simulink model "gm_uz_pmsm_model_9ph_vnl"  (R2021a)
settings: Solver=FixedStepAuto  StartTime=0.0  StopTime=.5  RelTol=1e-3
PreLoadFcn:
  | uz_pmsm_model_init_parameter
undefined symbols (not defined in the file or in its folder): c, friction_coefficient, inertia, k_i_d, k_p_d, k_p_q, L_d, L_o1, L_o2, L_q, L_x1, L_x2, L_y1, L_y2, L_zero, polepair, psi_pm, R_1, static_friction_torque, ts
libraries: hdlmdlgenlib x220, hdlsllib x18, simulink x11, pid_lib x2
(part 4 of 4)

== system gm_uz_pmsm_model_9ph_vnl/uz_pmsm_model_9ph/Transformation/Divide2 ==
  In1 : Inport
  In2 : Inport  Port=2
  Divide2 : Product  Inputs=**  OutDataTypeStr=single  SampleTime=1e-08
  Out1 : Outport
  wires:
  Divide2/1 -> Out1/1
  In2/1 -> Divide2/2
  In1/1 -> Divide2/1

== system gm_uz_pmsm_model_9ph_vnl/uz_pmsm_model_9ph/Transformation/Divide3 ==
  In1 : Inport
  In2 : Inport  Port=2
  Divide3 : Product  Inputs=**  OutDataTypeStr=single  SampleTime=1e-08
  Out1 : Outport
  wires:
  Divide3/1 -> Out1/1
  In2/1 -> Divide3/2
  In1/1 -> Divide3/1

== system gm_uz_pmsm_model_9ph_vnl/uz_pmsm_model_9ph/Transformation/Transformation_MAC ==
  in0 : Inport  OutDataTypeStr=fixdt(1, 18, 19)  PortDimensions=[9 1]  SampleTime=1e-08
  in1 : Inport  Port=2  OutDataTypeStr=fixdt(1, 25, 12)  PortDimensions=[9]  SampleTime=1e-08
  globalSchedule : EnablePort  OutDataTypeStr=boolean
  PipelineRegister : Delay  DelayLength=double(8)  InitialCondition=0
  t : hdlsllib/HDL Operations/Multiply-Accumulate  opMode=Vector  initValueSetting=Dialog  initValue=0  initValueSetting2=Dialog  initValue2=0  initValueSetting3=Dialog  initValue3=0  num_samples=2  RndMeth2=Floor  RndMeth3=Floor  OutDataTypeStr=fixdt(1, 43, 31)  datatype2=Inherit: Inherit via back propagation  datatype3=Inherit: Inherit via back propagation  validOut=on  endInandOut=on  startOut=on  countOut=on  dim=-1  DoSatur=off  parallel=off
      settings: SourceProductBaseCode=SL
  out0 : Outport  OutDataTypeStr=fixdt(1, 43, 31)  SampleTime=1e-08  InitialOutput=0
  wires:
  t/1 -> PipelineRegister/1
  in1/1 -> t/2
  in0/1 -> t/1
  PipelineRegister/1 -> out0/1

== system gm_uz_pmsm_model_9ph_vnl/uz_pmsm_model_9ph/Transformation/Transformation_MAC1 ==
  in0 : Inport  OutDataTypeStr=fixdt(1, 18, 19)  PortDimensions=[9 1]  SampleTime=1e-08
  in1 : Inport  Port=2  OutDataTypeStr=fixdt(1, 25, 12)  PortDimensions=[9]  SampleTime=1e-08
  globalSchedule : EnablePort  OutDataTypeStr=boolean
  PipelineRegister : Delay  DelayLength=double(8)  InitialCondition=0
  t : hdlsllib/HDL Operations/Multiply-Accumulate  opMode=Vector  initValueSetting=Dialog  initValue=0  initValueSetting2=Dialog  initValue2=0  initValueSetting3=Dialog  initValue3=0  num_samples=2  RndMeth2=Floor  RndMeth3=Floor  OutDataTypeStr=fixdt(1, 43, 31)  datatype2=Inherit: Inherit via back propagation  datatype3=Inherit: Inherit via back propagation  validOut=on  endInandOut=on  startOut=on  countOut=on  dim=-1  DoSatur=off  parallel=off
      settings: SourceProductBaseCode=SL
  out0 : Outport  OutDataTypeStr=fixdt(1, 43, 31)  SampleTime=1e-08  InitialOutput=0
  wires:
  t/1 -> PipelineRegister/1
  in1/1 -> t/2
  in0/1 -> t/1
  PipelineRegister/1 -> out0/1

== system gm_uz_pmsm_model_9ph_vnl/uz_pmsm_model_9ph/Transformation/Transformation_MAC2 ==
  in0 : Inport  OutDataTypeStr=fixdt(1, 18, 19)  PortDimensions=[9 1]  SampleTime=1e-08
  in1 : Inport  Port=2  OutDataTypeStr=fixdt(1, 25, 12)  PortDimensions=[9]  SampleTime=1e-08
  globalSchedule : EnablePort  OutDataTypeStr=boolean
  PipelineRegister : Delay  DelayLength=double(8)  InitialCondition=0
  t : hdlsllib/HDL Operations/Multiply-Accumulate  opMode=Vector  initValueSetting=Dialog  initValue=0  initValueSetting2=Dialog  initValue2=0  initValueSetting3=Dialog  initValue3=0  num_samples=2  RndMeth2=Floor  RndMeth3=Floor  OutDataTypeStr=fixdt(1, 43, 31)  datatype2=Inherit: Inherit via back propagation  datatype3=Inherit: Inherit via back propagation  validOut=on  endInandOut=on  startOut=on  countOut=on  dim=-1  DoSatur=off  parallel=off
      settings: SourceProductBaseCode=SL
  out0 : Outport  OutDataTypeStr=fixdt(1, 43, 31)  SampleTime=1e-08  InitialOutput=0
  wires:
  t/1 -> PipelineRegister/1
  in1/1 -> t/2
  in0/1 -> t/1
  PipelineRegister/1 -> out0/1

== system gm_uz_pmsm_model_9ph_vnl/uz_pmsm_model_9ph/Transformation/Transformation_MAC3 ==
  in0 : Inport  OutDataTypeStr=fixdt(1, 18, 19)  PortDimensions=[9 1]  SampleTime=1e-08
  in1 : Inport  Port=2  OutDataTypeStr=fixdt(1, 25, 12)  PortDimensions=[9]  SampleTime=1e-08
  globalSchedule : EnablePort  OutDataTypeStr=boolean
  PipelineRegister : Delay  DelayLength=double(8)  InitialCondition=0
  t : hdlsllib/HDL Operations/Multiply-Accumulate  opMode=Vector  initValueSetting=Dialog  initValue=0  initValueSetting2=Dialog  initValue2=0  initValueSetting3=Dialog  initValue3=0  num_samples=2  RndMeth2=Floor  RndMeth3=Floor  OutDataTypeStr=fixdt(1, 43, 31)  datatype2=Inherit: Inherit via back propagation  datatype3=Inherit: Inherit via back propagation  validOut=on  endInandOut=on  startOut=on  countOut=on  dim=-1  DoSatur=off  parallel=off
      settings: SourceProductBaseCode=SL
  out0 : Outport  OutDataTypeStr=fixdt(1, 43, 31)  SampleTime=1e-08  InitialOutput=0
  wires:
  t/1 -> PipelineRegister/1
  in1/1 -> t/2
  in0/1 -> t/1
  PipelineRegister/1 -> out0/1

== system gm_uz_pmsm_model_9ph_vnl/uz_pmsm_model_9ph/Transformation/Transformation_MAC4 ==
  in0 : Inport  OutDataTypeStr=fixdt(1, 18, 19)  PortDimensions=[9 1]  SampleTime=1e-08
  in1 : Inport  Port=2  OutDataTypeStr=fixdt(1, 25, 12)  PortDimensions=[9]  SampleTime=1e-08
  globalSchedule : EnablePort  OutDataTypeStr=boolean
  PipelineRegister : Delay  DelayLength=double(8)  InitialCondition=0
  t : hdlsllib/HDL Operations/Multiply-Accumulate  opMode=Vector  initValueSetting=Dialog  initValue=0  initValueSetting2=Dialog  initValue2=0  initValueSetting3=Dialog  initValue3=0  num_samples=2  RndMeth2=Floor  RndMeth3=Floor  OutDataTypeStr=fixdt(1, 43, 31)  datatype2=Inherit: Inherit via back propagation  datatype3=Inherit: Inherit via back propagation  validOut=on  endInandOut=on  startOut=on  countOut=on  dim=-1  DoSatur=off  parallel=off
      settings: SourceProductBaseCode=SL
  out0 : Outport  OutDataTypeStr=fixdt(1, 43, 31)  SampleTime=1e-08  InitialOutput=0
  wires:
  t/1 -> PipelineRegister/1
  in1/1 -> t/2
  in0/1 -> t/1
  PipelineRegister/1 -> out0/1

== system gm_uz_pmsm_model_9ph_vnl/uz_pmsm_model_9ph/Transformation/Transformation_MAC5 ==
  in0 : Inport  OutDataTypeStr=fixdt(1, 18, 19)  PortDimensions=[9 1]  SampleTime=1e-08
  in1 : Inport  Port=2  OutDataTypeStr=fixdt(1, 25, 12)  PortDimensions=[9]  SampleTime=1e-08
  globalSchedule : EnablePort  OutDataTypeStr=boolean
  PipelineRegister : Delay  DelayLength=double(8)  InitialCondition=0
  t : hdlsllib/HDL Operations/Multiply-Accumulate  opMode=Vector  initValueSetting=Dialog  initValue=0  initValueSetting2=Dialog  initValue2=0  initValueSetting3=Dialog  initValue3=0  num_samples=2  RndMeth2=Floor  RndMeth3=Floor  OutDataTypeStr=fixdt(1, 43, 31)  datatype2=Inherit: Inherit via back propagation  datatype3=Inherit: Inherit via back propagation  validOut=on  endInandOut=on  startOut=on  countOut=on  dim=-1  DoSatur=off  parallel=off
      settings: SourceProductBaseCode=SL
  out0 : Outport  OutDataTypeStr=fixdt(1, 43, 31)  SampleTime=1e-08  InitialOutput=0
  wires:
  t/1 -> PipelineRegister/1
  in1/1 -> t/2
  in0/1 -> t/1
  PipelineRegister/1 -> out0/1

== system gm_uz_pmsm_model_9ph_vnl/uz_pmsm_model_9ph/Transformation/Transformation_MAC6 ==
  in0 : Inport  OutDataTypeStr=fixdt(1, 18, 19)  PortDimensions=[9 1]  SampleTime=1e-08
  in1 : Inport  Port=2  OutDataTypeStr=fixdt(1, 25, 12)  PortDimensions=[9]  SampleTime=1e-08
  globalSchedule : EnablePort  OutDataTypeStr=boolean
  PipelineRegister : Delay  DelayLength=double(8)  InitialCondition=0
  t : hdlsllib/HDL Operations/Multiply-Accumulate  opMode=Vector  initValueSetting=Dialog  initValue=0  initValueSetting2=Dialog  initValue2=0  initValueSetting3=Dialog  initValue3=0  num_samples=2  RndMeth2=Floor  RndMeth3=Floor  OutDataTypeStr=fixdt(1, 43, 31)  datatype2=Inherit: Inherit via back propagation  datatype3=Inherit: Inherit via back propagation  validOut=on  endInandOut=on  startOut=on  countOut=on  dim=-1  DoSatur=off  parallel=off
      settings: SourceProductBaseCode=SL
  out0 : Outport  OutDataTypeStr=fixdt(1, 43, 31)  SampleTime=1e-08  InitialOutput=0
  wires:
  t/1 -> PipelineRegister/1
  in1/1 -> t/2
  in0/1 -> t/1
  PipelineRegister/1 -> out0/1

== system gm_uz_pmsm_model_9ph_vnl/uz_pmsm_model_9ph/Transformation/Transformation_MAC7 ==
  in0 : Inport  OutDataTypeStr=fixdt(1, 18, 19)  PortDimensions=[9 1]  SampleTime=1e-08
  in1 : Inport  Port=2  OutDataTypeStr=fixdt(1, 25, 12)  PortDimensions=[9]  SampleTime=1e-08
  globalSchedule : EnablePort  OutDataTypeStr=boolean
  PipelineRegister : Delay  DelayLength=double(8)  InitialCondition=0
  t : hdlsllib/HDL Operations/Multiply-Accumulate  opMode=Vector  initValueSetting=Dialog  initValue=0  initValueSetting2=Dialog  initValue2=0  initValueSetting3=Dialog  initValue3=0  num_samples=2  RndMeth2=Floor  RndMeth3=Floor  OutDataTypeStr=fixdt(1, 43, 31)  datatype2=Inherit: Inherit via back propagation  datatype3=Inherit: Inherit via back propagation  validOut=on  endInandOut=on  startOut=on  countOut=on  dim=-1  DoSatur=off  parallel=off
      settings: SourceProductBaseCode=SL
  out0 : Outport  OutDataTypeStr=fixdt(1, 43, 31)  SampleTime=1e-08  InitialOutput=0
  wires:
  t/1 -> PipelineRegister/1
  in1/1 -> t/2
  in0/1 -> t/1
  PipelineRegister/1 -> out0/1

== system gm_uz_pmsm_model_9ph_vnl/uz_pmsm_model_9ph/Transformation/Transformation_MAC8 ==
  in0 : Inport  OutDataTypeStr=fixdt(1, 18, 19)  PortDimensions=[9 1]  SampleTime=1e-08
  in1 : Inport  Port=2  OutDataTypeStr=fixdt(1, 25, 12)  PortDimensions=[9]  SampleTime=1e-08
  globalSchedule : EnablePort  OutDataTypeStr=boolean
  PipelineRegister : Delay  DelayLength=double(8)  InitialCondition=0
  t : hdlsllib/HDL Operations/Multiply-Accumulate  opMode=Vector  initValueSetting=Dialog  initValue=0  initValueSetting2=Dialog  initValue2=0  initValueSetting3=Dialog  initValue3=0  num_samples=2  RndMeth2=Floor  RndMeth3=Floor  OutDataTypeStr=fixdt(1, 43, 31)  datatype2=Inherit: Inherit via back propagation  datatype3=Inherit: Inherit via back propagation  validOut=on  endInandOut=on  startOut=on  countOut=on  dim=-1  DoSatur=off  parallel=off
      settings: SourceProductBaseCode=SL
  out0 : Outport  OutDataTypeStr=fixdt(1, 43, 31)  SampleTime=1e-08  InitialOutput=0
  wires:
  t/1 -> PipelineRegister/1
  in1/1 -> t/2
  in0/1 -> t/1
  PipelineRegister/1 -> out0/1

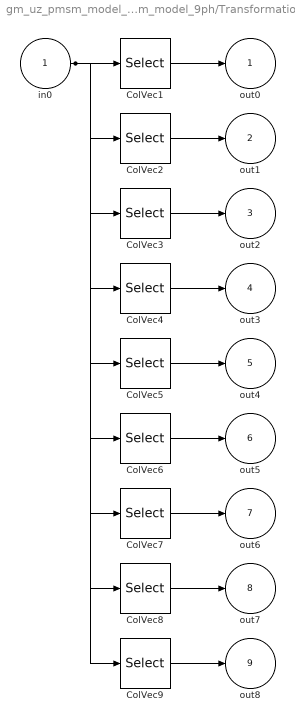
== system gm_uz_pmsm_model_9ph_vnl/uz_pmsm_model_9ph/Transformation/t3 ==
  in0 : Inport
  ColVec1 : Selector  NumberOfDimensions=2  IndexOptions=Select all,Index vector (dialog)  Indices=1,1  OutputSizes=1,1
  ColVec2 : Selector  NumberOfDimensions=2  IndexOptions=Select all,Index vector (dialog)  Indices=1,2  OutputSizes=1,1
  ColVec3 : Selector  NumberOfDimensions=2  IndexOptions=Select all,Index vector (dialog)  Indices=1,3  OutputSizes=1,1
  ColVec4 : Selector  NumberOfDimensions=2  IndexOptions=Select all,Index vector (dialog)  Indices=1,4  OutputSizes=1,1
  ColVec5 : Selector  NumberOfDimensions=2  IndexOptions=Select all,Index vector (dialog)  Indices=1,5  OutputSizes=1,1
  ColVec6 : Selector  NumberOfDimensions=2  IndexOptions=Select all,Index vector (dialog)  Indices=1,6  OutputSizes=1,1
  ColVec7 : Selector  NumberOfDimensions=2  IndexOptions=Select all,Index vector (dialog)  Indices=1,7  OutputSizes=1,1
  ColVec8 : Selector  NumberOfDimensions=2  IndexOptions=Select all,Index vector (dialog)  Indices=1,8  OutputSizes=1,1
  ColVec9 : Selector  NumberOfDimensions=2  IndexOptions=Select all,Index vector (dialog)  Indices=1,9  OutputSizes=1,1
  out0 : Outport
  out1 : Outport  Port=2
  out2 : Outport  Port=3
  out3 : Outport  Port=4
  out4 : Outport  Port=5
  out5 : Outport  Port=6
  out6 : Outport  Port=7
  out7 : Outport  Port=8
  out8 : Outport  Port=9
  wires:
  ColVec9/1 -> out8/1
  ColVec8/1 -> out7/1
  ColVec7/1 -> out6/1
  ColVec6/1 -> out5/1
  ColVec5/1 -> out4/1
  ColVec4/1 -> out3/1
  ColVec3/1 -> out2/1
  ColVec2/1 -> out1/1
  ColVec1/1 -> out0/1
  in0/1 -> ColVec9/1, ColVec8/1, ColVec7/1, ColVec6/1, ColVec5/1, ColVec4/1, ColVec3/1, ColVec2/1, ColVec1/1

== system gm_uz_pmsm_model_9ph_vnl/uz_pmsm_model_9ph/Transformation1/Add ==
  In1 : Inport
  In2 : Inport  Port=2
  Add : Sum  Inputs=+-  OutDataTypeStr=single  SampleTime=1e-08
  Out1 : Outport
  wires:
  Add/1 -> Out1/1
  In2/1 -> Add/2
  In1/1 -> Add/1

== system gm_uz_pmsm_model_9ph_vnl/uz_pmsm_model_9ph/Transformation1/Add1 ==
  In1 : Inport
  In2 : Inport  Port=2
  Add1 : Sum  OutDataTypeStr=single  SampleTime=1e-08
  Out1 : Outport
  wires:
  Add1/1 -> Out1/1
  In2/1 -> Add1/2
  In1/1 -> Add1/1

== system gm_uz_pmsm_model_9ph_vnl/uz_pmsm_model_9ph/Transformation1/Data Type Conversion28 ==
  In1 : Inport
  Data Type Conversion28 : DataTypeConversion  OutDataTypeStr=fixdt(1, 25, 12)  RndMeth=Nearest  SampleTime=1e-08
  Out1 : Outport
  wires:
  Data Type Conversion28/1 -> Out1/1
  In1/1 -> Data Type Conversion28/1

== system gm_uz_pmsm_model_9ph_vnl/uz_pmsm_model_9ph/Transformation1/Divide ==
  In1 : Inport
  In2 : Inport  Port=2
  Divide : Product  Inputs=**  OutDataTypeStr=single  SampleTime=1e-08
  Out1 : Outport
  wires:
  Divide/1 -> Out1/1
  In2/1 -> Divide/2
  In1/1 -> Divide/1

== system gm_uz_pmsm_model_9ph_vnl/uz_pmsm_model_9ph/Transformation1/Divide1 ==
  In1 : Inport
  In2 : Inport  Port=2
  Divide1 : Product  Inputs=**  OutDataTypeStr=single  SampleTime=1e-08
  Out1 : Outport
  wires:
  Divide1/1 -> Out1/1
  In2/1 -> Divide1/2
  In1/1 -> Divide1/1

== system gm_uz_pmsm_model_9ph_vnl/uz_pmsm_model_9ph/Transformation1/Divide2 ==
  In1 : Inport
  In2 : Inport  Port=2
  Divide2 : Product  Inputs=**  OutDataTypeStr=single  SampleTime=1e-08
  Out1 : Outport
  wires:
  Divide2/1 -> Out1/1
  In2/1 -> Divide2/2
  In1/1 -> Divide2/1

== system gm_uz_pmsm_model_9ph_vnl/uz_pmsm_model_9ph/Transformation1/Divide3 ==
  In1 : Inport
  In2 : Inport  Port=2
  Divide3 : Product  Inputs=**  OutDataTypeStr=single  SampleTime=1e-08
  Out1 : Outport
  wires:
  Divide3/1 -> Out1/1
  In2/1 -> Divide3/2
  In1/1 -> Divide3/1

== system gm_uz_pmsm_model_9ph_vnl/uz_pmsm_model_9ph/Transformation1/Transformation1_MAC ==
  in0 : Inport  OutDataTypeStr=fixdt(1, 18, 16)  PortDimensions=[9 1]  SampleTime=1e-08
  in1 : Inport  Port=2  OutDataTypeStr=fixdt(1, 25, 12)  PortDimensions=[9]  SampleTime=1e-08
  globalSchedule : EnablePort  OutDataTypeStr=boolean
  PipelineRegister : Delay  DelayLength=double(8)  InitialCondition=0
  t : hdlsllib/HDL Operations/Multiply-Accumulate  opMode=Vector  initValueSetting=Dialog  initValue=0  initValueSetting2=Dialog  initValue2=0  initValueSetting3=Dialog  initValue3=0  num_samples=2  RndMeth2=Floor  RndMeth3=Floor  OutDataTypeStr=fixdt(1, 43, 28)  datatype2=Inherit: Inherit via back propagation  datatype3=Inherit: Inherit via back propagation  validOut=on  endInandOut=on  startOut=on  countOut=on  dim=-1  DoSatur=off  parallel=off
      settings: SourceProductBaseCode=SL
  out0 : Outport  OutDataTypeStr=fixdt(1, 43, 28)  SampleTime=1e-08  InitialOutput=0
  wires:
  t/1 -> PipelineRegister/1
  in1/1 -> t/2
  in0/1 -> t/1
  PipelineRegister/1 -> out0/1

== system gm_uz_pmsm_model_9ph_vnl/uz_pmsm_model_9ph/Transformation1/Transformation1_MAC1 ==
  in0 : Inport  OutDataTypeStr=fixdt(1, 18, 16)  PortDimensions=[9 1]  SampleTime=1e-08
  in1 : Inport  Port=2  OutDataTypeStr=fixdt(1, 25, 12)  PortDimensions=[9]  SampleTime=1e-08
  globalSchedule : EnablePort  OutDataTypeStr=boolean
  PipelineRegister : Delay  DelayLength=double(8)  InitialCondition=0
  t : hdlsllib/HDL Operations/Multiply-Accumulate  opMode=Vector  initValueSetting=Dialog  initValue=0  initValueSetting2=Dialog  initValue2=0  initValueSetting3=Dialog  initValue3=0  num_samples=2  RndMeth2=Floor  RndMeth3=Floor  OutDataTypeStr=fixdt(1, 43, 28)  datatype2=Inherit: Inherit via back propagation  datatype3=Inherit: Inherit via back propagation  validOut=on  endInandOut=on  startOut=on  countOut=on  dim=-1  DoSatur=off  parallel=off
      settings: SourceProductBaseCode=SL
  out0 : Outport  OutDataTypeStr=fixdt(1, 43, 28)  SampleTime=1e-08  InitialOutput=0
  wires:
  t/1 -> PipelineRegister/1
  in1/1 -> t/2
  in0/1 -> t/1
  PipelineRegister/1 -> out0/1

== system gm_uz_pmsm_model_9ph_vnl/uz_pmsm_model_9ph/Transformation1/Transformation1_MAC2 ==
  in0 : Inport  OutDataTypeStr=fixdt(1, 18, 16)  PortDimensions=[9 1]  SampleTime=1e-08
  in1 : Inport  Port=2  OutDataTypeStr=fixdt(1, 25, 12)  PortDimensions=[9]  SampleTime=1e-08
  globalSchedule : EnablePort  OutDataTypeStr=boolean
  PipelineRegister : Delay  DelayLength=double(8)  InitialCondition=0
  t : hdlsllib/HDL Operations/Multiply-Accumulate  opMode=Vector  initValueSetting=Dialog  initValue=0  initValueSetting2=Dialog  initValue2=0  initValueSetting3=Dialog  initValue3=0  num_samples=2  RndMeth2=Floor  RndMeth3=Floor  OutDataTypeStr=fixdt(1, 43, 28)  datatype2=Inherit: Inherit via back propagation  datatype3=Inherit: Inherit via back propagation  validOut=on  endInandOut=on  startOut=on  countOut=on  dim=-1  DoSatur=off  parallel=off
      settings: SourceProductBaseCode=SL
  out0 : Outport  OutDataTypeStr=fixdt(1, 43, 28)  SampleTime=1e-08  InitialOutput=0
  wires:
  t/1 -> PipelineRegister/1
  in1/1 -> t/2
  in0/1 -> t/1
  PipelineRegister/1 -> out0/1

== system gm_uz_pmsm_model_9ph_vnl/uz_pmsm_model_9ph/Transformation1/Transformation1_MAC3 ==
  in0 : Inport  OutDataTypeStr=fixdt(1, 18, 16)  PortDimensions=[9 1]  SampleTime=1e-08
  in1 : Inport  Port=2  OutDataTypeStr=fixdt(1, 25, 12)  PortDimensions=[9]  SampleTime=1e-08
  globalSchedule : EnablePort  OutDataTypeStr=boolean
  PipelineRegister : Delay  DelayLength=double(8)  InitialCondition=0
  t : hdlsllib/HDL Operations/Multiply-Accumulate  opMode=Vector  initValueSetting=Dialog  initValue=0  initValueSetting2=Dialog  initValue2=0  initValueSetting3=Dialog  initValue3=0  num_samples=2  RndMeth2=Floor  RndMeth3=Floor  OutDataTypeStr=fixdt(1, 43, 28)  datatype2=Inherit: Inherit via back propagation  datatype3=Inherit: Inherit via back propagation  validOut=on  endInandOut=on  startOut=on  countOut=on  dim=-1  DoSatur=off  parallel=off
      settings: SourceProductBaseCode=SL
  out0 : Outport  OutDataTypeStr=fixdt(1, 43, 28)  SampleTime=1e-08  InitialOutput=0
  wires:
  t/1 -> PipelineRegister/1
  in1/1 -> t/2
  in0/1 -> t/1
  PipelineRegister/1 -> out0/1

== system gm_uz_pmsm_model_9ph_vnl/uz_pmsm_model_9ph/Transformation1/Transformation1_MAC4 ==
  in0 : Inport  OutDataTypeStr=fixdt(1, 18, 16)  PortDimensions=[9 1]  SampleTime=1e-08
  in1 : Inport  Port=2  OutDataTypeStr=fixdt(1, 25, 12)  PortDimensions=[9]  SampleTime=1e-08
  globalSchedule : EnablePort  OutDataTypeStr=boolean
  PipelineRegister : Delay  DelayLength=double(8)  InitialCondition=0
  t : hdlsllib/HDL Operations/Multiply-Accumulate  opMode=Vector  initValueSetting=Dialog  initValue=0  initValueSetting2=Dialog  initValue2=0  initValueSetting3=Dialog  initValue3=0  num_samples=2  RndMeth2=Floor  RndMeth3=Floor  OutDataTypeStr=fixdt(1, 43, 28)  datatype2=Inherit: Inherit via back propagation  datatype3=Inherit: Inherit via back propagation  validOut=on  endInandOut=on  startOut=on  countOut=on  dim=-1  DoSatur=off  parallel=off
      settings: SourceProductBaseCode=SL
  out0 : Outport  OutDataTypeStr=fixdt(1, 43, 28)  SampleTime=1e-08  InitialOutput=0
  wires:
  t/1 -> PipelineRegister/1
  in1/1 -> t/2
  in0/1 -> t/1
  PipelineRegister/1 -> out0/1

== system gm_uz_pmsm_model_9ph_vnl/uz_pmsm_model_9ph/Transformation1/Transformation1_MAC5 ==
  in0 : Inport  OutDataTypeStr=fixdt(1, 18, 16)  PortDimensions=[9 1]  SampleTime=1e-08
  in1 : Inport  Port=2  OutDataTypeStr=fixdt(1, 25, 12)  PortDimensions=[9]  SampleTime=1e-08
  globalSchedule : EnablePort  OutDataTypeStr=boolean
  PipelineRegister : Delay  DelayLength=double(8)  InitialCondition=0
  t : hdlsllib/HDL Operations/Multiply-Accumulate  opMode=Vector  initValueSetting=Dialog  initValue=0  initValueSetting2=Dialog  initValue2=0  initValueSetting3=Dialog  initValue3=0  num_samples=2  RndMeth2=Floor  RndMeth3=Floor  OutDataTypeStr=fixdt(1, 43, 28)  datatype2=Inherit: Inherit via back propagation  datatype3=Inherit: Inherit via back propagation  validOut=on  endInandOut=on  startOut=on  countOut=on  dim=-1  DoSatur=off  parallel=off
      settings: SourceProductBaseCode=SL
  out0 : Outport  OutDataTypeStr=fixdt(1, 43, 28)  SampleTime=1e-08  InitialOutput=0
  wires:
  t/1 -> PipelineRegister/1
  in1/1 -> t/2
  in0/1 -> t/1
  PipelineRegister/1 -> out0/1

== system gm_uz_pmsm_model_9ph_vnl/uz_pmsm_model_9ph/Transformation1/Transformation1_MAC6 ==
  in0 : Inport  OutDataTypeStr=fixdt(1, 18, 16)  PortDimensions=[9 1]  SampleTime=1e-08
  in1 : Inport  Port=2  OutDataTypeStr=fixdt(1, 25, 12)  PortDimensions=[9]  SampleTime=1e-08
  globalSchedule : EnablePort  OutDataTypeStr=boolean
  PipelineRegister : Delay  DelayLength=double(8)  InitialCondition=0
  t : hdlsllib/HDL Operations/Multiply-Accumulate  opMode=Vector  initValueSetting=Dialog  initValue=0  initValueSetting2=Dialog  initValue2=0  initValueSetting3=Dialog  initValue3=0  num_samples=2  RndMeth2=Floor  RndMeth3=Floor  OutDataTypeStr=fixdt(1, 43, 28)  datatype2=Inherit: Inherit via back propagation  datatype3=Inherit: Inherit via back propagation  validOut=on  endInandOut=on  startOut=on  countOut=on  dim=-1  DoSatur=off  parallel=off
      settings: SourceProductBaseCode=SL
  out0 : Outport  OutDataTypeStr=fixdt(1, 43, 28)  SampleTime=1e-08  InitialOutput=0
  wires:
  t/1 -> PipelineRegister/1
  in1/1 -> t/2
  in0/1 -> t/1
  PipelineRegister/1 -> out0/1

== system gm_uz_pmsm_model_9ph_vnl/uz_pmsm_model_9ph/Transformation1/Transformation1_MAC7 ==
  in0 : Inport  OutDataTypeStr=fixdt(1, 18, 16)  PortDimensions=[9 1]  SampleTime=1e-08
  in1 : Inport  Port=2  OutDataTypeStr=fixdt(1, 25, 12)  PortDimensions=[9]  SampleTime=1e-08
  globalSchedule : EnablePort  OutDataTypeStr=boolean
  PipelineRegister : Delay  DelayLength=double(8)  InitialCondition=0
  t : hdlsllib/HDL Operations/Multiply-Accumulate  opMode=Vector  initValueSetting=Dialog  initValue=0  initValueSetting2=Dialog  initValue2=0  initValueSetting3=Dialog  initValue3=0  num_samples=2  RndMeth2=Floor  RndMeth3=Floor  OutDataTypeStr=fixdt(1, 43, 28)  datatype2=Inherit: Inherit via back propagation  datatype3=Inherit: Inherit via back propagation  validOut=on  endInandOut=on  startOut=on  countOut=on  dim=-1  DoSatur=off  parallel=off
      settings: SourceProductBaseCode=SL
  out0 : Outport  OutDataTypeStr=fixdt(1, 43, 28)  SampleTime=1e-08  InitialOutput=0
  wires:
  t/1 -> PipelineRegister/1
  in1/1 -> t/2
  in0/1 -> t/1
  PipelineRegister/1 -> out0/1

== system gm_uz_pmsm_model_9ph_vnl/uz_pmsm_model_9ph/Transformation1/Transformation1_MAC8 ==
  in0 : Inport  OutDataTypeStr=fixdt(1, 18, 16)  PortDimensions=[9 1]  SampleTime=1e-08
  in1 : Inport  Port=2  OutDataTypeStr=fixdt(1, 25, 12)  PortDimensions=[9]  SampleTime=1e-08
  globalSchedule : EnablePort  OutDataTypeStr=boolean
  PipelineRegister : Delay  DelayLength=double(8)  InitialCondition=0
  t : hdlsllib/HDL Operations/Multiply-Accumulate  opMode=Vector  initValueSetting=Dialog  initValue=0  initValueSetting2=Dialog  initValue2=0  initValueSetting3=Dialog  initValue3=0  num_samples=2  RndMeth2=Floor  RndMeth3=Floor  OutDataTypeStr=fixdt(1, 43, 28)  datatype2=Inherit: Inherit via back propagation  datatype3=Inherit: Inherit via back propagation  validOut=on  endInandOut=on  startOut=on  countOut=on  dim=-1  DoSatur=off  parallel=off
      settings: SourceProductBaseCode=SL
  out0 : Outport  OutDataTypeStr=fixdt(1, 43, 28)  SampleTime=1e-08  InitialOutput=0
  wires:
  t/1 -> PipelineRegister/1
  in1/1 -> t/2
  in0/1 -> t/1
  PipelineRegister/1 -> out0/1

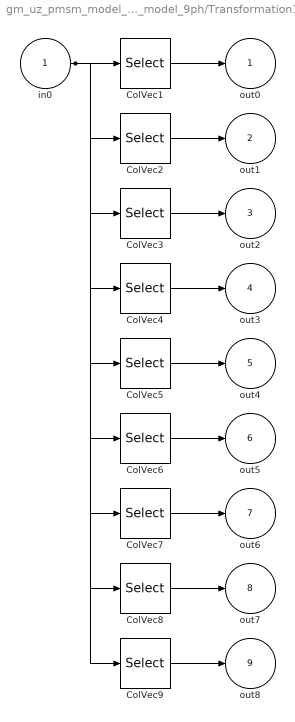
== system gm_uz_pmsm_model_9ph_vnl/uz_pmsm_model_9ph/Transformation1/t3 ==
  in0 : Inport
  ColVec1 : Selector  NumberOfDimensions=2  IndexOptions=Select all,Index vector (dialog)  Indices=1,1  OutputSizes=1,1
  ColVec2 : Selector  NumberOfDimensions=2  IndexOptions=Select all,Index vector (dialog)  Indices=1,2  OutputSizes=1,1
  ColVec3 : Selector  NumberOfDimensions=2  IndexOptions=Select all,Index vector (dialog)  Indices=1,3  OutputSizes=1,1
  ColVec4 : Selector  NumberOfDimensions=2  IndexOptions=Select all,Index vector (dialog)  Indices=1,4  OutputSizes=1,1
  ColVec5 : Selector  NumberOfDimensions=2  IndexOptions=Select all,Index vector (dialog)  Indices=1,5  OutputSizes=1,1
  ColVec6 : Selector  NumberOfDimensions=2  IndexOptions=Select all,Index vector (dialog)  Indices=1,6  OutputSizes=1,1
  ColVec7 : Selector  NumberOfDimensions=2  IndexOptions=Select all,Index vector (dialog)  Indices=1,7  OutputSizes=1,1
  ColVec8 : Selector  NumberOfDimensions=2  IndexOptions=Select all,Index vector (dialog)  Indices=1,8  OutputSizes=1,1
  ColVec9 : Selector  NumberOfDimensions=2  IndexOptions=Select all,Index vector (dialog)  Indices=1,9  OutputSizes=1,1
  out0 : Outport
  out1 : Outport  Port=2
  out2 : Outport  Port=3
  out3 : Outport  Port=4
  out4 : Outport  Port=5
  out5 : Outport  Port=6
  out6 : Outport  Port=7
  out7 : Outport  Port=8
  out8 : Outport  Port=9
  wires:
  ColVec9/1 -> out8/1
  ColVec8/1 -> out7/1
  ColVec7/1 -> out6/1
  ColVec6/1 -> out5/1
  ColVec5/1 -> out4/1
  ColVec4/1 -> out3/1
  ColVec3/1 -> out2/1
  ColVec2/1 -> out1/1
  ColVec1/1 -> out0/1
  in0/1 -> ColVec9/1, ColVec8/1, ColVec7/1, ColVec6/1, ColVec5/1, ColVec4/1, ColVec3/1, ColVec2/1, ColVec1/1

== system gm_uz_pmsm_model_9ph_vnl/uz_pmsm_model_9ph_vnl/mechanical_system/integrator1 ==
  reset : Inport
  in : Inport  Port=2
  Delay1 : Delay  DelayLength=1  ExternalReset=Level
      settings: InputPortMap=u0,r5
  Gain : Gain  Gain=ts  OutDataTypeStr=double
  Sum3 : Sum  Inputs=|++  OutDataTypeStr=double
  outt : Outport
  wires:
  Delay1/1 -> outt/1, Sum3/2
  Sum3/1 -> Delay1/1
  reset/1 -> Delay1/2
  Gain/1 -> Sum3/1
  in/1 -> Gain/1

== system gm_uz_pmsm_model_9ph_vnl/uz_pmsm_model_9ph_vnl/pmsm/integrator ==
  in : Inport
  reset : Inport  Port=2
  Delay1 : Delay  DelayLength=1  ExternalReset=Level
      settings: InputPortMap=u0,r5
  Gain : Gain  Gain=ts  OutDataTypeStr=double
  Sum3 : Sum  Inputs=|++  OutDataTypeStr=double
  outt : Outport
  wires:
  Sum3/1 -> Delay1/1
  Delay1/1 -> Sum3/2, outt/1
  in/1 -> Gain/1
  Gain/1 -> Sum3/1
  reset/1 -> Delay1/2

== system gm_uz_pmsm_model_9ph_vnl/uz_pmsm_model_9ph_vnl/pmsm/integrator1 ==
  in : Inport
  reset : Inport  Port=2
  Delay1 : Delay  DelayLength=1  ExternalReset=Level
      settings: InputPortMap=u0,r5
  Gain : Gain  Gain=ts  OutDataTypeStr=double
  Sum3 : Sum  Inputs=|++  OutDataTypeStr=double
  outt : Outport
  wires:
  Sum3/1 -> Delay1/1
  Delay1/1 -> outt/1, Sum3/2
  reset/1 -> Delay1/2
  Gain/1 -> Sum3/1
  in/1 -> Gain/1

== system gm_uz_pmsm_model_9ph_vnl/uz_pmsm_model_9ph_vnl/pmsm/integrator2 ==
  in : Inport
  reset : Inport  Port=2
  Delay1 : Delay  DelayLength=1  ExternalReset=Level
      settings: InputPortMap=u0,r5
  Gain : Gain  Gain=ts  OutDataTypeStr=double
  Sum3 : Sum  Inputs=|++  OutDataTypeStr=double
  outt : Outport
  wires:
  Sum3/1 -> Delay1/1
  Delay1/1 -> outt/1, Sum3/2
  reset/1 -> Delay1/2
  Gain/1 -> Sum3/1
  in/1 -> Gain/1

== system gm_uz_pmsm_model_9ph_vnl/uz_pmsm_model_9ph_vnl/pmsm/integrator3 ==
  in : Inport
  reset : Inport  Port=2
  Delay1 : Delay  DelayLength=1  ExternalReset=Level
      settings: InputPortMap=u0,r5
  Gain : Gain  Gain=ts  OutDataTypeStr=double
  Sum3 : Sum  Inputs=|++  OutDataTypeStr=double
  outt : Outport
  wires:
  in/1 -> Gain/1
  Gain/1 -> Sum3/1
  reset/1 -> Delay1/2
  Delay1/1 -> Sum3/2, outt/1
  Sum3/1 -> Delay1/1

== system gm_uz_pmsm_model_9ph_vnl/uz_pmsm_model_9ph_vnl/pmsm/integrator4 ==
  in : Inport
  reset : Inport  Port=2
  Delay1 : Delay  DelayLength=1  ExternalReset=Level
      settings: InputPortMap=u0,r5
  Gain : Gain  Gain=ts  OutDataTypeStr=double
  Sum3 : Sum  Inputs=|++  OutDataTypeStr=double
  outt : Outport
  wires:
  Sum3/1 -> Delay1/1
  Delay1/1 -> outt/1, Sum3/2
  reset/1 -> Delay1/2
  Gain/1 -> Sum3/1
  in/1 -> Gain/1

== system gm_uz_pmsm_model_9ph_vnl/uz_pmsm_model_9ph_vnl/pmsm/integrator5 ==
  in : Inport
  reset : Inport  Port=2
  Delay1 : Delay  DelayLength=1  ExternalReset=Level
      settings: InputPortMap=u0,r5
  Gain : Gain  Gain=ts  OutDataTypeStr=double
  Sum3 : Sum  Inputs=|++  OutDataTypeStr=double
  outt : Outport
  wires:
  in/1 -> Gain/1
  Gain/1 -> Sum3/1
  reset/1 -> Delay1/2
  Delay1/1 -> Sum3/2, outt/1
  Sum3/1 -> Delay1/1

== system gm_uz_pmsm_model_9ph_vnl/uz_pmsm_model_9ph_vnl/pmsm/integrator6 ==
  in : Inport
  reset : Inport  Port=2
  Delay1 : Delay  DelayLength=1  ExternalReset=Level
      settings: InputPortMap=u0,r5
  Gain : Gain  Gain=ts  OutDataTypeStr=double
  Sum3 : Sum  Inputs=|++  OutDataTypeStr=double
  outt : Outport
  wires:
  Sum3/1 -> Delay1/1
  Delay1/1 -> outt/1, Sum3/2
  reset/1 -> Delay1/2
  Gain/1 -> Sum3/1
  in/1 -> Gain/1

== system gm_uz_pmsm_model_9ph_vnl/uz_pmsm_model_9ph_vnl/pmsm/integrator7 ==
  in : Inport
  reset : Inport  Port=2
  Delay1 : Delay  DelayLength=1  ExternalReset=Level
      settings: InputPortMap=u0,r5
  Gain : Gain  Gain=ts  OutDataTypeStr=double
  Sum3 : Sum  Inputs=|++  OutDataTypeStr=double
  outt : Outport
  wires:
  in/1 -> Gain/1
  Gain/1 -> Sum3/1
  reset/1 -> Delay1/2
  Delay1/1 -> Sum3/2, outt/1
  Sum3/1 -> Delay1/1

== system gm_uz_pmsm_model_9ph_vnl/uz_pmsm_model_9ph_vnl/pmsm/integrator8 ==
  in : Inport
  reset : Inport  Port=2
  Delay1 : Delay  DelayLength=1  ExternalReset=Level
      settings: InputPortMap=u0,r5
  Gain : Gain  Gain=ts  OutDataTypeStr=double
  Sum3 : Sum  Inputs=|++  OutDataTypeStr=double
  outt : Outport
  wires:
  Sum3/1 -> Delay1/1
  Delay1/1 -> outt/1, Sum3/2
  reset/1 -> Delay1/2
  Gain/1 -> Sum3/1
  in/1 -> Gain/1

== matlab function gm_uz_pmsm_model_9ph_vnl/Compare/Assert_output_currents_abc/RelErrCheck/RelativeErrorCheck  ==
  data: P input; y output; R input; ToleranceValue parameter double
% Check if the relative error of R with respect to P is below
% ToleranceValue
% P, R are floating-point
function y = relErrCheck(P,R, ToleranceValue)
    tol = ToleranceValue;
    sz = numel(P);
    assert(sz == numel(R), 'Inputs P and R have different sizes.');
    y = false(1, sz);

    for ii=1:sz
        if (isnan(P(ii)) || isnan(R(ii)))
            if (isnan(P(ii)) && isnan(R(ii)))
                y(ii) = true;
            end
        elseif (isinf(P(ii)) || isinf(R(ii)))
            y(ii) = (P(ii) == R(ii));
        elseif (P(ii) == 0)
            y(ii) = (R(ii) == 0);
        else
            absdiff = abs(P(ii) - R(ii));
            relerr = absdiff/abs(P(ii));
            y(ii) = (relerr <= tol);
        end
    end
end

== matlab function gm_uz_pmsm_model_9ph_vnl/Compare/Assert_output_general/RelErrCheck/RelativeErrorCheck  ==
  data: P input; y output; R input; ToleranceValue parameter double
% Check if the relative error of R with respect to P is below
% ToleranceValue
% P, R are floating-point
function y = relErrCheck(P,R, ToleranceValue)
    tol = ToleranceValue;
    sz = numel(P);
    assert(sz == numel(R), 'Inputs P and R have different sizes.');
    y = false(1, sz);

    for ii=1:sz
        if (isnan(P(ii)) || isnan(R(ii)))
            if (isnan(P(ii)) && isnan(R(ii)))
                y(ii) = true;
            end
        elseif (isinf(P(ii)) || isinf(R(ii)))
            y(ii) = (P(ii) == R(ii));
        elseif (P(ii) == 0)
            y(ii) = (R(ii) == 0);
        else
            absdiff = abs(P(ii) - R(ii));
            relerr = absdiff/abs(P(ii));
            y(ii) = (relerr <= tol);
        end
    end
end

== matlab function gm_uz_pmsm_model_9ph_vnl/Compare/Assert_output_currents_dq/RelErrCheck/RelativeErrorCheck  ==
  data: P input; y output; R input; ToleranceValue parameter double
% Check if the relative error of R with respect to P is below
% ToleranceValue
% P, R are floating-point
function y = relErrCheck(P,R, ToleranceValue)
    tol = ToleranceValue;
    sz = numel(P);
    assert(sz == numel(R), 'Inputs P and R have different sizes.');
    y = false(1, sz);

    for ii=1:sz
        if (isnan(P(ii)) || isnan(R(ii)))
            if (isnan(P(ii)) && isnan(R(ii)))
                y(ii) = true;
            end
        elseif (isinf(P(ii)) || isinf(R(ii)))
            y(ii) = (P(ii) == R(ii));
        elseif (P(ii) == 0)
            y(ii) = (R(ii) == 0);
        else
            absdiff = abs(P(ii) - R(ii));
            relerr = absdiff/abs(P(ii));
            y(ii) = (relerr <= tol);
        end
    end
end
